simulink model "auv"  (R2022b)
settings: Solver=VariableStepAuto  StartTime=0.0  StopTime=50  FixedStep=0.000025  RelTol=1e-3
InitFcn:
  | tavola3
undefined symbols (not defined in the file or in its folder): C_lq, C_lu, C_lw, C_qq, C_qu, C_qw, I, m
settings Model: Creator=Giovanni  LastModifiedBy=morel

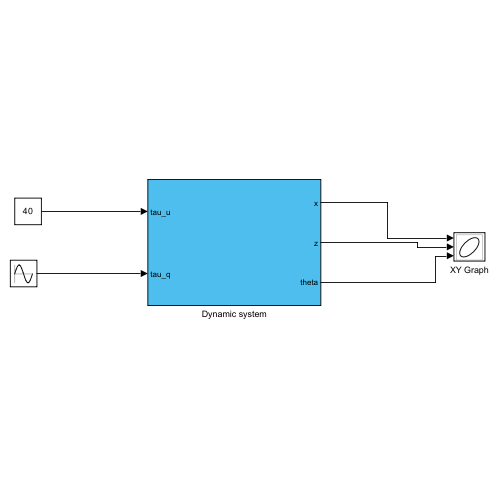
[thumbnail: Simulink's stored preview of the top-level diagram]
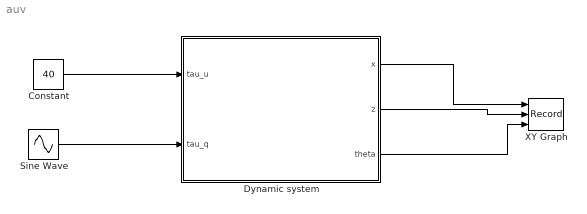
== system auv ==
  Constant : Constant  Value=40
  Dynamic system : Subsystem
  Sine Wave : Sin  Amplitude=2.2  Frequency=0.1969  SampleTime=0
  XY Graph : Record  FileSettingsInternal="{\"entries\":[{\"content\":{\"excelSettings\":{\"content\":{},\"type\":\"Streamout.ExcelSettings\"}},\"type\":\"Streamout.FileSettingStorage\",\"uuid\":\"e1367d25-f4f9-4769-be61-ba01c35a76b8\"}],\"packageUris\":[\"http://schema.mathworks.com/mf0/streamout_blocks/R2020a\"],\"version\":\"1.0\"}"  Layout=[1 1]  SignalsInternal="{\"entries\":[{\"content\":{\"signals\":[{\"content\":{\"blockPath\":[\"auv/XY Graph\"],\"channel\":[],\"dimensions\":[1],\"domain\":\"auv/XY Graph\",\"lineColor\":\"#a2142f\",\"plots\":[1],\"port\":1,\"sid\":[],\"signalID\":24,\"signalName\":\"Dynamic system:1\"},\"type\":\"RecordBlkView.Signal\",\"uuid\":\"8e98420e-07de-413b-bd8b-743d53131de1\"},{\"content\":{\"blockPath\":[\"auv/XY Graph\"],\"channel\":[],\"dimensions\":[1],\"domain\":\"auv/XY Graph\",\"lineColor\":\"#139fff\",\"plots\":[1],\"port\":2,\"sid\":[],\"signalID\":27,\"signalName\":\"Dynamic system:2\"},\"type\":\"RecordBlkView.Signal\",\"uuid\":\"bd925e29-cc18-482f-b9c9-1ee3220ccf55\"},{\"content\":{\"blockPath\":[\"auv/XY Graph\"],\"channel\":[],\"dimensions\":[1],\"domain\":\"auv/XY Graph\",\"lineColor\":\"#a2142f\",\"plots\":[],\"port\":3,\"sid\":[],\"signalID\":30,\"signalName\":\"Dynamic system:3\"},\"type\":\"RecordBlkView.Signal\",\"uuid\":\"ef33a519-5830-430b-ada9-a98bf7b6dc9b\"}]},\"type\":\"RecordBlkView.InputSignals\",\"uuid\":\"c5017561-b61e-49c5-8e44-6d946aedb9c2\"}],\"packageUris\":[\"http://schema.mathworks.com/mf0/streamout_blocks/R2020a\"],\"version\":\"1.0\"}"  VisualizationBindings="{\"xyplotplugin\":{\"info\":[{\"series\":[{\"bindingParametersList\":[{\"parameter\":\"X-Axis\",\"signalID\":24,\"signalName\":\"Dynamic system:1\"},{\"parameter\":\"Y-Axis\",\"signalID\":27,\"signalName\":\"Dynamic system:2\"}],\"seriesID\":43710}],\"subplotID\":1}]}}"  CompatibilityTag=XY
  wires:
  Constant/1 -> Dynamic system/1(tau_u)
  Sine Wave/1 -> Dynamic system/2(tau_q)
  Dynamic system/1(x) -> XY Graph/1
  Dynamic system/2(z) -> XY Graph/2
  Dynamic system/3(theta) -> XY Graph/3

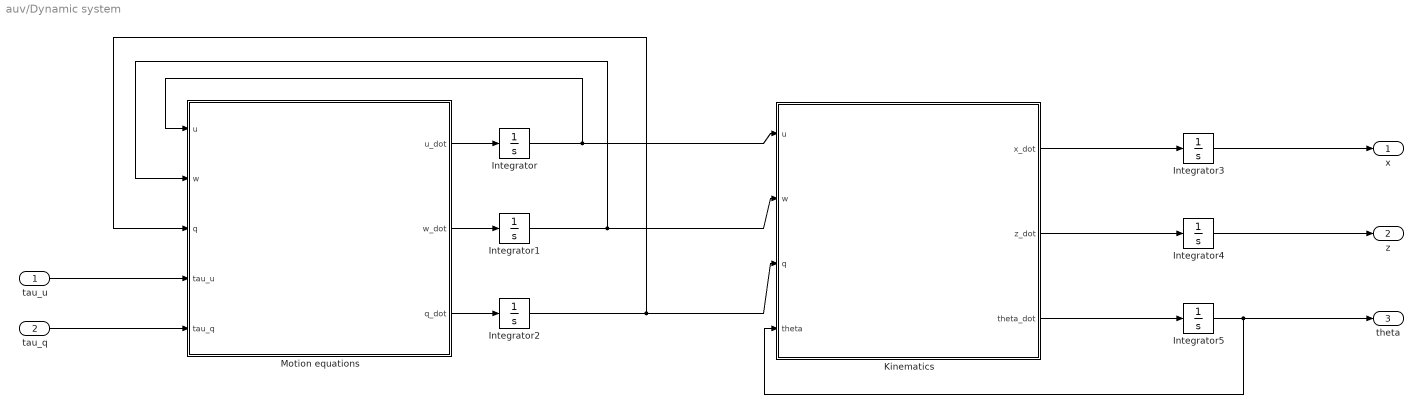
== system auv/Dynamic system ==
  tau_u : Inport
  tau_q : Inport  Port=2
  Integrator{,1..2,5} (4 alike) : Integrator
  Integrator3 : Integrator  InitialCondition=150
  Integrator4 : Integrator  InitialCondition=25
  Kinematics : MATLAB Function  TreatAsAtomicUnit=on
  Motion equations : MATLAB Function  TreatAsAtomicUnit=on
  x : Outport
  z : Outport  Port=2
  theta : Outport  Port=3
  wires:
  Integrator3/1 -> x/1
  Kinematics/2(z_dot) -> Integrator4/1
  Integrator/1 -> Motion equations/1(u), Kinematics/1(u)
  Integrator1/1 -> Motion equations/2(w), Kinematics/2(w)
  Motion equations/2(w_dot) -> Integrator1/1
  tau_u/1 -> Motion equations/4(tau_u)
  Integrator5/1 -> theta/1, Kinematics/4(theta)
  Motion equations/1(u_dot) -> Integrator/1
  Motion equations/3(q_dot) -> Integrator2/1
  Integrator2/1 -> Motion equations/3(q), Kinematics/3(q)
  Kinematics/3(theta_dot) -> Integrator5/1
  Kinematics/1(x_dot) -> Integrator3/1
  tau_q/1 -> Motion equations/5(tau_q)
  Integrator4/1 -> z/1

== matlab function auv/Dynamic system/Kinematics ==
  settings: updateMethod=CONTINUOUS
  data: u input; x_dot output; w input; q input; theta input; z_dot output; theta_dot output
function [x_dot, z_dot, theta_dot] = kinematics(u,w,q,theta)

 %% DEFINISCO PARAMETRI USATI NELLA FUNZIONE
    Rz = [cos(theta) sin(theta) 0   ; %
         -sin(theta) cos(theta) 0   ; % MATRICE DI ROTAZIONE ATTORNO ALL'ASSE Z
            0           0       1 ] ; % 
%% CAMBIO SISTEMA DI RIFERIMENTO DA TERNA BODY A SISTEMA FISSO     
    out = Rz*[u w q]';

%% FORNISCO IN USCITA LE SINGOLE COMPONENTI    
    x_dot     = out(1);
    z_dot     = out(2);
    theta_dot = out(3);

== matlab function auv/Dynamic system/Motion equations ==
  settings: updateMethod=CONTINUOUS
  data: u input; u_dot output; w input; q input; tau_u input; tau_q input; w_dot output; q_dot output; m parameter; I parameter; C_qu parameter; C_lu parameter; C_lw parameter; C_qw parameter; C_lq parameter; C_qq parameter
function [u_dot,w_dot,q_dot] = motion(u,w,q,tau_u,tau_q,m, I, C_qu, C_lu, C_lw, C_qw, C_lq, C_qq)

 % Inversione della dinamica del sistema per ricavare le accelerazioni,
 % portiamo le informazioni in forma matriciale per semplicità
    
    U = [u w q]';                               % Vettore velocità

    B = [m 0 0 ;
         0 m 0 ;                                % Matrice inerzia
         0 0 I];

    C = [  0     0   m*w ;                      %
           0     0  -m*u ;                      % Matrice coriolis
         -m*w   m*u   0 ];                      %

    F = [ C_lu+C_qu*abs(u)   0            0              ;  %
              0          C_lw+C_qw*abs(w) 0              ;  %   Matrice reistenza avanzamento
              0              0       C_lq + C_qq*abs(q) ];  %

    Q = [tau_u 0 tau_q]';                       % Vettore controllo

    
    O = B\(Q-C*U-F*U);                        % Inversione dinamica 
    
    u_dot=O(1);                                 
    w_dot=O(2);
    q_dot=O(3);

end
